simulink model "test"  (R2021a)
settings: Solver=VariableStepAuto  StartTime=0.0  StopTime=60000  RelTol=1e-3
undefined symbols (not defined in the file): Ion, Lithium
libraries: spsSeriesRLCBranchLib x25, spsBatteryLib x20, spsIGBTLib x20, spsIdealSwitchLib x10, spsDCVoltageSourceLib x5, spspowerguiLib x1
settings Model: SimulationMode=rapid-accelerator  Creator=jafar  LastModifiedBy=jafar

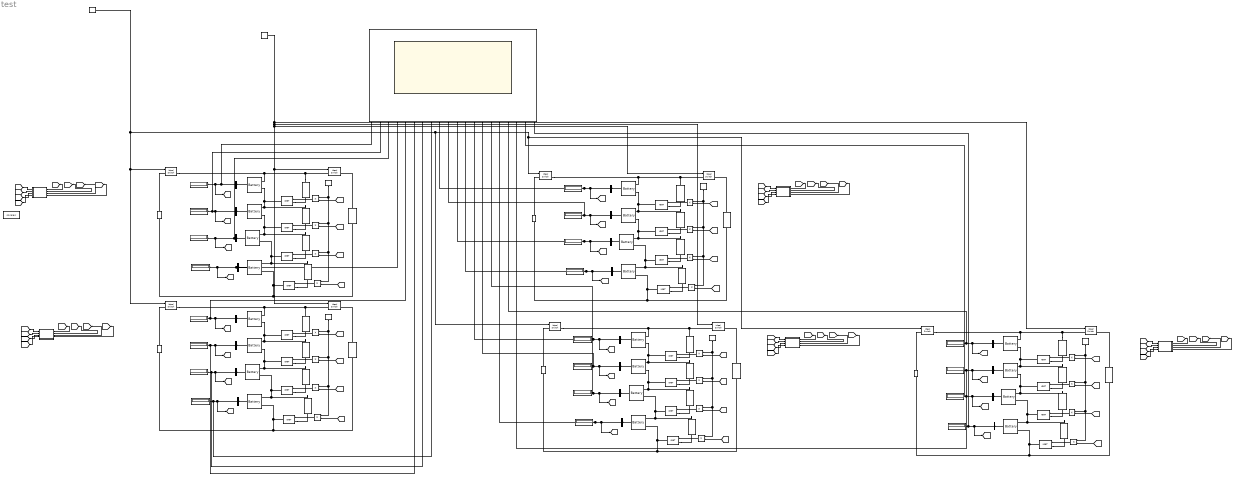
== system test ==
  Battery : spsBatteryLib/Battery  BatType=Lithium-Ion  ShowTempParam=off  ThermalPreset=no  ShowAgeParam=off  NomV=3.7  NomQ=30  SOC=20  Batt_Tr=30  PresetModel=on  MaxQ=30  MinV=2.775  FullV=4.3068  Dis_rate=13.0435  R=0.0012333  Normal_OP=27.1304  expZone="[3.9974      1.4739]"  current=[6.5 13 32.5]  Units=Time  Tci=20  NomT=20  T2=-30  MaxQ2=4.8  FullV2=7.1  Normal_OP2=5.655  expZone2="[6.58           1]"  Rca=0.6  ti=2000  Dp=0  Neq0=0  Tsim=1e6  Ta1=25  Qeol=5.4*0.9  Reol=0.013333*1.2  Char_age=[2.3478, 3]  Dis_age=[2.3478, 10]  N1=1500  N2=10500  N3=1000  N4=1400  Ta2=45  N5=950
  Battery1 : spsBatteryLib/Battery  BatType=Lithium-Ion  ShowTempParam=off  ThermalPreset=no  ShowAgeParam=off  NomV=3.7  NomQ=30  SOC=23  Batt_Tr=30  PresetModel=on  MaxQ=30  MinV=2.775  FullV=4.3068  Dis_rate=13.0435  R=0.0012333  Normal_OP=27.1304  expZone="[3.9974      1.4739]"  current=[6.5 13 32.5]  Units=Time  Tci=20  NomT=20  T2=-30  MaxQ2=4.8  FullV2=7.1  Normal_OP2=5.655  expZone2="[6.58           1]"  Rca=0.6  ti=2000  Dp=0  Neq0=0  Tsim=1e6  Ta1=25  Qeol=5.4*0.9  Reol=0.013333*1.2  Char_age=[2.3478, 3]  Dis_age=[2.3478, 10]  N1=1500  N2=10500  N3=1000  N4=1400  Ta2=45  N5=950
  Battery10 : spsBatteryLib/Battery  BatType=Lithium-Ion  ShowTempParam=off  ThermalPreset=no  ShowAgeParam=off  NomV=3.7  NomQ=30  SOC=60  Batt_Tr=30  PresetModel=on  MaxQ=30  MinV=2.775  FullV=4.3068  Dis_rate=13.0435  R=0.0012333  Normal_OP=27.1304  expZone="[3.9974      1.4739]"  current=[6.5 13 32.5]  Units=Time  Tci=20  NomT=20  T2=-30  MaxQ2=4.8  FullV2=7.1  Normal_OP2=5.655  expZone2="[6.58           1]"  Rca=0.6  ti=2000  Dp=0  Neq0=0  Tsim=1e6  Ta1=25  Qeol=5.4*0.9  Reol=0.013333*1.2  Char_age=[2.3478, 3]  Dis_age=[2.3478, 10]  N1=1500  N2=10500  N3=1000  N4=1400  Ta2=45  N5=950
  Battery11 : spsBatteryLib/Battery  BatType=Lithium-Ion  ShowTempParam=off  ThermalPreset=no  ShowAgeParam=off  NomV=3.7  NomQ=30  SOC=63  Batt_Tr=30  PresetModel=on  MaxQ=30  MinV=2.775  FullV=4.3068  Dis_rate=13.0435  R=0.0012333  Normal_OP=27.1304  expZone="[3.9974      1.4739]"  current=[6.5 13 32.5]  Units=Time  Tci=20  NomT=20  T2=-30  MaxQ2=4.8  FullV2=7.1  Normal_OP2=5.655  expZone2="[6.58           1]"  Rca=0.6  ti=2000  Dp=0  Neq0=0  Tsim=1e6  Ta1=25  Qeol=5.4*0.9  Reol=0.013333*1.2  Char_age=[2.3478, 3]  Dis_age=[2.3478, 10]  N1=1500  N2=10500  N3=1000  N4=1400  Ta2=45  N5=950
  Battery12 : spsBatteryLib/Battery  BatType=Lithium-Ion  ShowTempParam=off  ThermalPreset=no  ShowAgeParam=off  NomV=3.7  NomQ=30  SOC=66  Batt_Tr=30  PresetModel=on  MaxQ=30  MinV=2.775  FullV=4.3068  Dis_rate=13.0435  R=0.0012333  Normal_OP=27.1304  expZone="[3.9974      1.4739]"  current=[6.5 13 32.5]  Units=Time  Tci=20  NomT=20  T2=-30  MaxQ2=4.8  FullV2=7.1  Normal_OP2=5.655  expZone2="[6.58           1]"  Rca=0.6  ti=2000  Dp=0  Neq0=0  Tsim=1e6  Ta1=25  Qeol=5.4*0.9  Reol=0.013333*1.2  Char_age=[2.3478, 3]  Dis_age=[2.3478, 10]  N1=1500  N2=10500  N3=1000  N4=1400  Ta2=45  N5=950
  Battery13 : spsBatteryLib/Battery  BatType=Lithium-Ion  ShowTempParam=off  ThermalPreset=no  ShowAgeParam=off  NomV=3.7  NomQ=30  SOC=69  Batt_Tr=30  PresetModel=on  MaxQ=30  MinV=2.775  FullV=4.3068  Dis_rate=13.0435  R=0.0012333  Normal_OP=27.1304  expZone="[3.9974      1.4739]"  current=[6.5 13 32.5]  Units=Time  Tci=20  NomT=20  T2=-30  MaxQ2=4.8  FullV2=7.1  Normal_OP2=5.655  expZone2="[6.58           1]"  Rca=0.6  ti=2000  Dp=0  Neq0=0  Tsim=1e6  Ta1=25  Qeol=5.4*0.9  Reol=0.013333*1.2  Char_age=[2.3478, 3]  Dis_age=[2.3478, 10]  N1=1500  N2=10500  N3=1000  N4=1400  Ta2=45  N5=950
  Battery14 : spsBatteryLib/Battery  BatType=Lithium-Ion  ShowTempParam=off  ThermalPreset=no  ShowAgeParam=off  NomV=3.7  NomQ=30  SOC=72  Batt_Tr=30  PresetModel=on  MaxQ=30  MinV=2.775  FullV=4.3068  Dis_rate=13.0435  R=0.0012333  Normal_OP=27.1304  expZone="[3.9974      1.4739]"  current=[6.5 13 32.5]  Units=Time  Tci=20  NomT=20  T2=-30  MaxQ2=4.8  FullV2=7.1  Normal_OP2=5.655  expZone2="[6.58           1]"  Rca=0.6  ti=2000  Dp=0  Neq0=0  Tsim=1e6  Ta1=25  Qeol=5.4*0.9  Reol=0.013333*1.2  Char_age=[2.3478, 3]  Dis_age=[2.3478, 10]  N1=1500  N2=10500  N3=1000  N4=1400  Ta2=45  N5=950
  Battery15 : spsBatteryLib/Battery  BatType=Lithium-Ion  ShowTempParam=off  ThermalPreset=no  ShowAgeParam=off  NomV=3.7  NomQ=30  SOC=75  Batt_Tr=30  PresetModel=on  MaxQ=30  MinV=2.775  FullV=4.3068  Dis_rate=13.0435  R=0.0012333  Normal_OP=27.1304  expZone="[3.9974      1.4739]"  current=[6.5 13 32.5]  Units=Time  Tci=20  NomT=20  T2=-30  MaxQ2=4.8  FullV2=7.1  Normal_OP2=5.655  expZone2="[6.58           1]"  Rca=0.6  ti=2000  Dp=0  Neq0=0  Tsim=1e6  Ta1=25  Qeol=5.4*0.9  Reol=0.013333*1.2  Char_age=[2.3478, 3]  Dis_age=[2.3478, 10]  N1=1500  N2=10500  N3=1000  N4=1400  Ta2=45  N5=950
  Battery16 : spsBatteryLib/Battery  BatType=Lithium-Ion  ShowTempParam=off  ThermalPreset=no  ShowAgeParam=off  NomV=3.7  NomQ=30  SOC=78  Batt_Tr=30  PresetModel=on  MaxQ=30  MinV=2.775  FullV=4.3068  Dis_rate=13.0435  R=0.0012333  Normal_OP=27.1304  expZone="[3.9974      1.4739]"  current=[6.5 13 32.5]  Units=Time  Tci=20  NomT=20  T2=-30  MaxQ2=4.8  FullV2=7.1  Normal_OP2=5.655  expZone2="[6.58           1]"  Rca=0.6  ti=2000  Dp=0  Neq0=0  Tsim=1e6  Ta1=25  Qeol=5.4*0.9  Reol=0.013333*1.2  Char_age=[2.3478, 3]  Dis_age=[2.3478, 10]  N1=1500  N2=10500  N3=1000  N4=1400  Ta2=45  N5=950
  Battery17 : spsBatteryLib/Battery  BatType=Lithium-Ion  ShowTempParam=off  ThermalPreset=no  ShowAgeParam=off  NomV=3.7  NomQ=30  SOC=32  Batt_Tr=30  PresetModel=on  MaxQ=30  MinV=2.775  FullV=4.3068  Dis_rate=13.0435  R=0.0012333  Normal_OP=27.1304  expZone="[3.9974      1.4739]"  current=[6.5 13 32.5]  Units=Time  Tci=20  NomT=20  T2=-30  MaxQ2=4.8  FullV2=7.1  Normal_OP2=5.655  expZone2="[6.58           1]"  Rca=0.6  ti=2000  Dp=0  Neq0=0  Tsim=1e6  Ta1=25  Qeol=5.4*0.9  Reol=0.013333*1.2  Char_age=[2.3478, 3]  Dis_age=[2.3478, 10]  N1=1500  N2=10500  N3=1000  N4=1400  Ta2=45  N5=950
  Battery18 : spsBatteryLib/Battery  BatType=Lithium-Ion  ShowTempParam=off  ThermalPreset=no  ShowAgeParam=off  NomV=3.7  NomQ=30  SOC=35  Batt_Tr=30  PresetModel=on  MaxQ=30  MinV=2.775  FullV=4.3068  Dis_rate=13.0435  R=0.0012333  Normal_OP=27.1304  expZone="[3.9974      1.4739]"  current=[6.5 13 32.5]  Units=Time  Tci=20  NomT=20  T2=-30  MaxQ2=4.8  FullV2=7.1  Normal_OP2=5.655  expZone2="[6.58           1]"  Rca=0.6  ti=2000  Dp=0  Neq0=0  Tsim=1e6  Ta1=25  Qeol=5.4*0.9  Reol=0.013333*1.2  Char_age=[2.3478, 3]  Dis_age=[2.3478, 10]  N1=1500  N2=10500  N3=1000  N4=1400  Ta2=45  N5=950
  Battery19 : spsBatteryLib/Battery  BatType=Lithium-Ion  ShowTempParam=off  ThermalPreset=no  ShowAgeParam=off  NomV=3.7  NomQ=30  SOC=38  Batt_Tr=30  PresetModel=on  MaxQ=30  MinV=2.775  FullV=4.3068  Dis_rate=13.0435  R=0.0012333  Normal_OP=27.1304  expZone="[3.9974      1.4739]"  current=[6.5 13 32.5]  Units=Time  Tci=20  NomT=20  T2=-30  MaxQ2=4.8  FullV2=7.1  Normal_OP2=5.655  expZone2="[6.58           1]"  Rca=0.6  ti=2000  Dp=0  Neq0=0  Tsim=1e6  Ta1=25  Qeol=5.4*0.9  Reol=0.013333*1.2  Char_age=[2.3478, 3]  Dis_age=[2.3478, 10]  N1=1500  N2=10500  N3=1000  N4=1400  Ta2=45  N5=950
  Battery2 : spsBatteryLib/Battery  BatType=Lithium-Ion  ShowTempParam=off  ThermalPreset=no  ShowAgeParam=off  NomV=3.7  NomQ=30  SOC=26  Batt_Tr=30  PresetModel=on  MaxQ=30  MinV=2.775  FullV=4.3068  Dis_rate=13.0435  R=0.0012333  Normal_OP=27.1304  expZone="[3.9974      1.4739]"  current=[6.5 13 32.5]  Units=Time  Tci=20  NomT=20  T2=-30  MaxQ2=4.8  FullV2=7.1  Normal_OP2=5.655  expZone2="[6.58           1]"  Rca=0.6  ti=2000  Dp=0  Neq0=0  Tsim=1e6  Ta1=25  Qeol=5.4*0.9  Reol=0.013333*1.2  Char_age=[2.3478, 3]  Dis_age=[2.3478, 10]  N1=1500  N2=10500  N3=1000  N4=1400  Ta2=45  N5=950
  Battery3 : spsBatteryLib/Battery  BatType=Lithium-Ion  ShowTempParam=off  ThermalPreset=no  ShowAgeParam=off  NomV=3.7  NomQ=30  SOC=29  Batt_Tr=30  PresetModel=on  MaxQ=30  MinV=2.775  FullV=4.3068  Dis_rate=13.0435  R=0.0012333  Normal_OP=27.1304  expZone="[3.9974      1.4739]"  current=[6.5 13 32.5]  Units=Time  Tci=20  NomT=20  T2=-30  MaxQ2=4.8  FullV2=7.1  Normal_OP2=5.655  expZone2="[6.58           1]"  Rca=0.6  ti=2000  Dp=0  Neq0=0  Tsim=1e6  Ta1=25  Qeol=5.4*0.9  Reol=0.013333*1.2  Char_age=[2.3478, 3]  Dis_age=[2.3478, 10]  N1=1500  N2=10500  N3=1000  N4=1400  Ta2=45  N5=950
  Battery4 : spsBatteryLib/Battery  BatType=Lithium-Ion  ShowTempParam=off  ThermalPreset=no  ShowAgeParam=off  NomV=3.7  NomQ=30  SOC=42  Batt_Tr=30  PresetModel=on  MaxQ=30  MinV=2.775  FullV=4.3068  Dis_rate=13.0435  R=0.0012333  Normal_OP=27.1304  expZone="[3.9974      1.4739]"  current=[6.5 13 32.5]  Units=Time  Tci=20  NomT=20  T2=-30  MaxQ2=4.8  FullV2=7.1  Normal_OP2=5.655  expZone2="[6.58           1]"  Rca=0.6  ti=2000  Dp=0  Neq0=0  Tsim=1e6  Ta1=25  Qeol=5.4*0.9  Reol=0.013333*1.2  Char_age=[2.3478, 3]  Dis_age=[2.3478, 10]  N1=1500  N2=10500  N3=1000  N4=1400  Ta2=45  N5=950
  Battery5 : spsBatteryLib/Battery  BatType=Lithium-Ion  ShowTempParam=off  ThermalPreset=no  ShowAgeParam=off  NomV=3.7  NomQ=30  SOC=45  Batt_Tr=30  PresetModel=on  MaxQ=30  MinV=2.775  FullV=4.3068  Dis_rate=13.0435  R=0.0012333  Normal_OP=27.1304  expZone="[3.9974      1.4739]"  current=[6.5 13 32.5]  Units=Time  Tci=20  NomT=20  T2=-30  MaxQ2=4.8  FullV2=7.1  Normal_OP2=5.655  expZone2="[6.58           1]"  Rca=0.6  ti=2000  Dp=0  Neq0=0  Tsim=1e6  Ta1=25  Qeol=5.4*0.9  Reol=0.013333*1.2  Char_age=[2.3478, 3]  Dis_age=[2.3478, 10]  N1=1500  N2=10500  N3=1000  N4=1400  Ta2=45  N5=950
  Battery6 : spsBatteryLib/Battery  BatType=Lithium-Ion  ShowTempParam=off  ThermalPreset=no  ShowAgeParam=off  NomV=3.7  NomQ=30  SOC=48  Batt_Tr=30  PresetModel=on  MaxQ=30  MinV=2.775  FullV=4.3068  Dis_rate=13.0435  R=0.0012333  Normal_OP=27.1304  expZone="[3.9974      1.4739]"  current=[6.5 13 32.5]  Units=Time  Tci=20  NomT=20  T2=-30  MaxQ2=4.8  FullV2=7.1  Normal_OP2=5.655  expZone2="[6.58           1]"  Rca=0.6  ti=2000  Dp=0  Neq0=0  Tsim=1e6  Ta1=25  Qeol=5.4*0.9  Reol=0.013333*1.2  Char_age=[2.3478, 3]  Dis_age=[2.3478, 10]  N1=1500  N2=10500  N3=1000  N4=1400  Ta2=45  N5=950
  Battery7 : spsBatteryLib/Battery  BatType=Lithium-Ion  ShowTempParam=off  ThermalPreset=no  ShowAgeParam=off  NomV=3.7  NomQ=30  SOC=51  Batt_Tr=30  PresetModel=on  MaxQ=30  MinV=2.775  FullV=4.3068  Dis_rate=13.0435  R=0.0012333  Normal_OP=27.1304  expZone="[3.9974      1.4739]"  current=[6.5 13 32.5]  Units=Time  Tci=20  NomT=20  T2=-30  MaxQ2=4.8  FullV2=7.1  Normal_OP2=5.655  expZone2="[6.58           1]"  Rca=0.6  ti=2000  Dp=0  Neq0=0  Tsim=1e6  Ta1=25  Qeol=5.4*0.9  Reol=0.013333*1.2  Char_age=[2.3478, 3]  Dis_age=[2.3478, 10]  N1=1500  N2=10500  N3=1000  N4=1400  Ta2=45  N5=950
  Battery8 : spsBatteryLib/Battery  BatType=Lithium-Ion  ShowTempParam=off  ThermalPreset=no  ShowAgeParam=off  NomV=3.7  NomQ=30  SOC=54  Batt_Tr=30  PresetModel=on  MaxQ=30  MinV=2.775  FullV=4.3068  Dis_rate=13.0435  R=0.0012333  Normal_OP=27.1304  expZone="[3.9974      1.4739]"  current=[6.5 13 32.5]  Units=Time  Tci=20  NomT=20  T2=-30  MaxQ2=4.8  FullV2=7.1  Normal_OP2=5.655  expZone2="[6.58           1]"  Rca=0.6  ti=2000  Dp=0  Neq0=0  Tsim=1e6  Ta1=25  Qeol=5.4*0.9  Reol=0.013333*1.2  Char_age=[2.3478, 3]  Dis_age=[2.3478, 10]  N1=1500  N2=10500  N3=1000  N4=1400  Ta2=45  N5=950
  Battery9 : spsBatteryLib/Battery  BatType=Lithium-Ion  ShowTempParam=off  ThermalPreset=no  ShowAgeParam=off  NomV=3.7  NomQ=30  SOC=57  Batt_Tr=30  PresetModel=on  MaxQ=30  MinV=2.775  FullV=4.3068  Dis_rate=13.0435  R=0.0012333  Normal_OP=27.1304  expZone="[3.9974      1.4739]"  current=[6.5 13 32.5]  Units=Time  Tci=20  NomT=20  T2=-30  MaxQ2=4.8  FullV2=7.1  Normal_OP2=5.655  expZone2="[6.58           1]"  Rca=0.6  ti=2000  Dp=0  Neq0=0  Tsim=1e6  Ta1=25  Qeol=5.4*0.9  Reol=0.013333*1.2  Char_age=[2.3478, 3]  Dis_age=[2.3478, 10]  N1=1500  N2=10500  N3=1000  N4=1400  Ta2=45  N5=950
  Bus Selector{,1..19} (20 alike) : BusSelector  OutputSignals=SOC (%)
  Constant{2..3,5,8,11,14} (6 alike) : Constant
  Constant13 : Constant  Value=0
  DC Voltage Source{,1..4} (5 alike) : spsDCVoltageSourceLib/DC Voltage Source  Amplitude=16.8  Measurements=None
  Display{,1..19} (20 alike) : Display
  IGBT{,1..19} (20 alike) : spsIGBTLib/IGBT  Ron=0.001  Lon=0  Vf=1  Tf=1e-6  Tt=2e-6  IC=0  Rs=1e5  Cs=inf  Measurements=off
  Ideal Switch{,1..9} (10 alike) : spsIdealSwitchLib/Ideal Switch  Ron=0.001  Lon=0  IC=0  Rs=1e5  Cs=inf  Measurements=on
  MATLAB Function : MATLAB Function  TreatAsAtomicUnit=on
  MATLAB Function1 : MATLAB Function  TreatAsAtomicUnit=on
  MATLAB Function2 : MATLAB Function  TreatAsAtomicUnit=on
  MATLAB Function3 : MATLAB Function  TreatAsAtomicUnit=on
  MATLAB Function4 : MATLAB Function  TreatAsAtomicUnit=on
  Product{,1..19} (20 alike) : Product
  Scope : Scope  NumInputPorts=20
  Series RLC Branch{,1..24} (25 alike) : spsSeriesRLCBranchLib/Series RLC Branch  LConnTagsString=__new0  RConnTagsString=__new0  BranchType=R  Resistance=1  Inductance=1e-3  SetiL0=off  InitialCurrent=0  Capacitance=1e-6  Setx0=off  InitialVoltage=0  Measurements=None
  powergui : spspowerguiLib/powergui  Priority=1  SimulationMode=Continuous  SampleTime=50e-6  frequency=60  Iterations=50  frequencyindice=0  Pbase=100e6  ErrMax=1e-4  UnitsV=kV  UnitsW=MW  buscounter=0  FunctionMessages=off  echomessages=off  EnableUseOfTLC=off  CurrentSourceSwitches=off  DisableSnubberDevices=off  DisableRonSwitches=off  DisableVfSwitches=off  DisplayEquations=off  AutomaticDiscreteSolvers=off  SolverType=Tustin/Backward Euler (TBE)  Interpol=off  ExternalGateDelay=off  methode=off  Ts=100  x0status=blocks  SPID=on  SwTol=0  HookPort=off  NonlinearTolerance=1e-4  nMaxIteration=100  ContinueOnMaxIteration=off  RestoreLinks=warning  ResistiveCurrentMeasurement=off  Frange=[0:2:500]  Ylog=off  Xlog=on  ShowGrid=off  save=off  variable=ZData  structure=0  ZoomFFT=off  StartTime=0.0  cycles=1  DisplayStyle=1  fundamental=60  FreqAxis=off  MaxFrequency=1000  frequencyindicesteady=1  RmsSteady=1  display=off
  wires:
  [g3] -> Product2/2
  Battery/1 -> Bus Selector/1
  Product2/1 -> IGBT/1
  [g2] -> Product1/2
  Bus Selector1/1 -> [SoC2], Display1/1, Scope/2  "<SOC (%)>"
  Product1/1 -> IGBT1/1
  [g1] -> Product/2
  Product/1 -> IGBT2/1
  Battery2/1 -> Bus Selector2/1
  Battery1/1 -> Bus Selector1/1
  Bus Selector/1 -> Display/1, [SoC1], Scope/1  "<SOC (%)>"
  Bus Selector2/1 -> Display2/1, [SoC3], Scope/3  "<SOC (%)>"
  Bus Selector3/1 -> Display3/1, [SoC4], Scope/4  "<SOC (%)>"
  Battery3/1 -> Bus Selector3/1
  Product3/1 -> IGBT3/1
  Constant2/1 -> Product/1, Product1/1, Product3/1, Product2/1
  [g4] -> Product3/2
  [SoC3] -> MATLAB Function/3(u3)
  [SoC2] -> MATLAB Function/2(u2)
  [SoC1] -> MATLAB Function/1(u1)
  MATLAB Function/2(g2) -> [g2]
  MATLAB Function/3(g3) -> [g3]
  MATLAB Function/1(g1) -> [g1]
  [SoC4] -> MATLAB Function/4(u4)
  MATLAB Function/4(g4) -> [g4]
  MATLAB Function1/2(g2) -> [g6]
  [SoC5] -> MATLAB Function1/1(u1)
  [SoC6] -> MATLAB Function1/2(u2)
  [SoC7] -> MATLAB Function1/3(u3)
  MATLAB Function1/3(g3) -> [g7]
  Battery7/1 -> Bus Selector7/1
  Product7/1 -> IGBT7/1
  Bus Selector7/1 -> [SoC8], Scope/8, Display7/1  "<SOC (%)>"
  MATLAB Function1/4(g4) -> [g8]
  Bus Selector6/1 -> [SoC7], Scope/7, Display6/1  "<SOC (%)>"
  Bus Selector4/1 -> [SoC5], Scope/5, Display4/1  "<SOC (%)>"
  Battery5/1 -> Bus Selector5/1
  [SoC8] -> MATLAB Function1/4(u4)
  Battery6/1 -> Bus Selector6/1
  [g5] -> Product4/2
  Product5/1 -> IGBT5/1
  MATLAB Function1/1(g1) -> [g5]
  Bus Selector5/1 -> [SoC6], Scope/6, Display5/1  "<SOC (%)>"
  [g6] -> Product5/2
  Battery4/1 -> Bus Selector4/1
  Constant5/1 -> Product4/1, Product5/1, Product7/1, Product6/1
  [g8] -> Product7/2
  Product6/1 -> IGBT4/1
  [g7] -> Product6/2
  Product4/1 -> IGBT6/1
  MATLAB Function2/2(g2) -> [g10]
  [SoC9] -> MATLAB Function2/1(u1)
  [SoC10] -> MATLAB Function2/2(u2)
  [SoC11] -> MATLAB Function2/3(u3)
  MATLAB Function2/3(g3) -> [g11]
  Battery11/1 -> Bus Selector11/1
  Product11/1 -> IGBT11/1
  Bus Selector11/1 -> [SoC12], Scope/12, Display11/1  "<SOC (%)>"
  MATLAB Function2/4(g4) -> [g12]
  Bus Selector10/1 -> [SoC11], Scope/11, Display10/1  "<SOC (%)>"
  Bus Selector8/1 -> [SoC9], Scope/9, Display8/1  "<SOC (%)>"
  Battery9/1 -> Bus Selector9/1
  [SoC12] -> MATLAB Function2/4(u4)
  Battery10/1 -> Bus Selector10/1
  [g9] -> Product8/2
  Product9/1 -> IGBT9/1
  MATLAB Function2/1(g1) -> [g9]
  Bus Selector9/1 -> [SoC10], Scope/10, Display9/1  "<SOC (%)>"
  [g10] -> Product9/2
  Battery8/1 -> Bus Selector8/1
  Constant8/1 -> Product8/1, Product9/1, Product11/1, Product10/1
  [g12] -> Product11/2
  Product10/1 -> IGBT8/1
  [g11] -> Product10/2
  Product8/1 -> IGBT10/1
  MATLAB Function3/2(g2) -> [g14]
  [SoC13] -> MATLAB Function3/1(u1)
  [SoC14] -> MATLAB Function3/2(u2)
  [SoC15] -> MATLAB Function3/3(u3)
  MATLAB Function3/3(g3) -> [g15]
  Battery15/1 -> Bus Selector15/1
  Product15/1 -> IGBT15/1
  Bus Selector15/1 -> [SoC16], Scope/16, Display15/1  "<SOC (%)>"
  MATLAB Function3/4(g4) -> [g16]
  Bus Selector14/1 -> [SoC15], Scope/15, Display14/1  "<SOC (%)>"
  Bus Selector12/1 -> [SoC13], Scope/13, Display12/1  "<SOC (%)>"
  Battery13/1 -> Bus Selector13/1
  [SoC16] -> MATLAB Function3/4(u4)
  Battery14/1 -> Bus Selector14/1
  [g13] -> Product12/2
  Product13/1 -> IGBT13/1
  MATLAB Function3/1(g1) -> [g13]
  Bus Selector13/1 -> [SoC14], Scope/14, Display13/1  "<SOC (%)>"
  [g14] -> Product13/2
  Battery12/1 -> Bus Selector12/1
  Constant11/1 -> Product12/1, Product13/1, Product15/1, Product14/1
  [g16] -> Product15/2
  Product14/1 -> IGBT12/1
  Constant13/1 -> Ideal Switch7/1, Ideal Switch5/1, Ideal Switch3/1, Ideal Switch1/1, Ideal Switch9/1
  [g15] -> Product14/2
  Product12/1 -> IGBT14/1
  MATLAB Function4/2(g2) -> [g18]
  MATLAB Function4/4(g4) -> [g20]
  Product16/1 -> IGBT18/1
  Product19/1 -> IGBT19/1
  Product18/1 -> IGBT16/1
  Constant3/1 -> Ideal Switch6/1, Ideal Switch8/1, Ideal Switch4/1, Ideal Switch2/1, Ideal Switch/1
  [SoC18] -> MATLAB Function4/2(u2)
  Battery19/1 -> Bus Selector19/1
  Battery17/1 -> Bus Selector17/1
  Bus Selector16/1 -> [SoC17], Scope/17, Display16/1  "<SOC (%)>"
  [g20] -> Product19/2
  Bus Selector18/1 -> [SoC19], Scope/19, Display18/1  "<SOC (%)>"
  MATLAB Function4/3(g3) -> [g19]
  Bus Selector17/1 -> [SoC18], Scope/18, Display17/1  "<SOC (%)>"
  [SoC17] -> MATLAB Function4/1(u1)
  MATLAB Function4/1(g1) -> [g17]
  Product17/1 -> IGBT17/1
  Battery18/1 -> Bus Selector18/1
  Constant14/1 -> Product16/1, Product17/1, Product19/1, Product18/1
  Battery16/1 -> Bus Selector16/1
  [SoC19] -> MATLAB Function4/3(u3)
  [g17] -> Product16/2
  Bus Selector19/1 -> [SoC20], Scope/20, Display19/1  "<SOC (%)>"
  [g18] -> Product17/2
  [g19] -> Product18/2
  [SoC20] -> MATLAB Function4/4(u4)
  connections:
  Series RLC Branch4/LConn1 -- Battery3/LConn1 -- Battery2/LConn2 -- IGBT/RConn1
  Battery1/LConn1 -- Battery/LConn2 -- IGBT2/RConn1 -- Series RLC Branch1/LConn1
  Series RLC Branch2/LConn1 -- Ideal Switch1/LConn1 -- Battery/LConn1 -- Ideal Switch/RConn1
  Battery2/LConn1 -- Battery1/LConn2 -- IGBT1/RConn1 -- Series RLC Branch/LConn1
  IGBT1/LConn1 -- Series RLC Branch1/RConn1
  IGBT/LConn1 -- Series RLC Branch/RConn1
  Series RLC Branch3/LConn1 -- Ideal Switch1/RConn1
  Ideal Switch/LConn1 -- DC Voltage Source/RConn1
  IGBT2/LConn1 -- Series RLC Branch2/RConn1
  Series RLC Branch3/RConn1 -- DC Voltage Source/LConn1 -- IGBT3/RConn1 -- Battery3/LConn2
  IGBT3/LConn1 -- Series RLC Branch4/RConn1
  Battery6/LConn1 -- Battery5/LConn2 -- IGBT5/RConn1 -- Series RLC Branch5/LConn1
  DC Voltage Source1/LConn1 -- Series RLC Branch8/RConn1 -- IGBT7/RConn1 -- Battery7/LConn2
  Battery5/LConn1 -- Battery4/LConn2 -- IGBT6/RConn1 -- Series RLC Branch6/LConn1
  Ideal Switch2/RConn1 -- Battery4/LConn1 -- Ideal Switch3/LConn1 -- Series RLC Branch7/LConn1
  IGBT4/RConn1 -- Battery6/LConn2 -- Battery7/LConn1 -- Series RLC Branch9/LConn1
  IGBT7/LConn1 -- Series RLC Branch9/RConn1
  IGBT6/LConn1 -- Series RLC Branch7/RConn1
  IGBT5/LConn1 -- Series RLC Branch6/RConn1
  Ideal Switch2/LConn1 -- DC Voltage Source1/RConn1
  IGBT4/LConn1 -- Series RLC Branch5/RConn1
  Series RLC Branch8/LConn1 -- Ideal Switch3/RConn1
  Battery10/LConn1 -- Battery9/LConn2 -- IGBT9/RConn1 -- Series RLC Branch10/LConn1
  DC Voltage Source2/LConn1 -- Series RLC Branch13/RConn1 -- IGBT11/RConn1 -- Battery11/LConn2
  Battery9/LConn1 -- Battery8/LConn2 -- IGBT10/RConn1 -- Series RLC Branch11/LConn1
  Ideal Switch4/RConn1 -- Battery8/LConn1 -- Ideal Switch5/LConn1 -- Series RLC Branch12/LConn1
  IGBT8/RConn1 -- Battery10/LConn2 -- Battery11/LConn1 -- Series RLC Branch14/LConn1
  IGBT11/LConn1 -- Series RLC Branch14/RConn1
  IGBT10/LConn1 -- Series RLC Branch12/RConn1
  IGBT9/LConn1 -- Series RLC Branch11/RConn1
  Ideal Switch4/LConn1 -- DC Voltage Source2/RConn1
  IGBT8/LConn1 -- Series RLC Branch10/RConn1
  Series RLC Branch13/LConn1 -- Ideal Switch5/RConn1
  Battery14/LConn1 -- Battery13/LConn2 -- IGBT13/RConn1 -- Series RLC Branch15/LConn1
  DC Voltage Source3/LConn1 -- Series RLC Branch18/RConn1 -- IGBT15/RConn1 -- Battery15/LConn2
  Battery13/LConn1 -- Battery12/LConn2 -- IGBT14/RConn1 -- Series RLC Branch16/LConn1
  Ideal Switch6/RConn1 -- Battery12/LConn1 -- Ideal Switch7/LConn1 -- Series RLC Branch17/LConn1
  IGBT12/RConn1 -- Battery14/LConn2 -- Battery15/LConn1 -- Series RLC Branch19/LConn1
  IGBT15/LConn1 -- Series RLC Branch19/RConn1
  IGBT14/LConn1 -- Series RLC Branch17/RConn1
  IGBT13/LConn1 -- Series RLC Branch16/RConn1
  Ideal Switch6/LConn1 -- DC Voltage Source3/RConn1
  IGBT12/LConn1 -- Series RLC Branch15/RConn1
  Series RLC Branch18/LConn1 -- Ideal Switch7/RConn1
  DC Voltage Source4/LConn1 -- Series RLC Branch23/RConn1 -- IGBT19/RConn1 -- Battery19/LConn2
  Battery18/LConn1 -- Battery17/LConn2 -- IGBT17/RConn1 -- Series RLC Branch20/LConn1
  Battery17/LConn1 -- Series RLC Branch21/LConn1 -- Battery16/LConn2 -- IGBT18/RConn1
  Series RLC Branch22/LConn1 -- Ideal Switch9/LConn1 -- Battery16/LConn1 -- Ideal Switch8/RConn1
  Series RLC Branch24/LConn1 -- Battery19/LConn1 -- Battery18/LConn2 -- IGBT16/RConn1
  IGBT17/LConn1 -- Series RLC Branch21/RConn1
  IGBT16/LConn1 -- Series RLC Branch20/RConn1
  Ideal Switch8/LConn1 -- DC Voltage Source4/RConn1
  IGBT18/LConn1 -- Series RLC Branch22/RConn1
  IGBT19/LConn1 -- Series RLC Branch24/RConn1
  Series RLC Branch23/LConn1 -- Ideal Switch9/RConn1

== matlab function test/MATLAB Function1 ==
  data: u1 input; g1 output; u2 input; u3 input; g2 output; g3 output; u4 input; g4 output
function [g1,g2,g3,g4] = fcn(u1,u2,u3,u4)

u1 = u1*1000;
u2 = u2*1000;
u3 = u3*1000;
u4 = u4*1000;

u1 = int32(u1);
u2 = int32(u2);
u3 = int32(u3);
u4 = int32(u4);

if u1>u2||u1>u3||u1>u4
    g1 = 1;
else
    g1 = 0;
end
    
if u2>u1||u2>u3||u2>u4
    g2 = 1;
else
    g2 = 0;
end

if u3>u1||u3>u2||u2>u4
    g3 = 1;
else
    g3 = 0;
end
if u4>u1||u4>u2||u4>u3
    g4 = 1;
else
    g4 = 0;
end

end

== matlab function test/MATLAB Function ==
  data: u1 input; g1 output; u2 input; u3 input; g2 output; g3 output; u4 input; g4 output
function [g1,g2,g3,g4] = fcn(u1,u2,u3,u4)

u1 = u1*1000;
u2 = u2*1000;
u3 = u3*1000;
u4 = u4*1000;

u1 = int32(u1);
u2 = int32(u2);
u3 = int32(u3);
u4 = int32(u4);

if u1>u2||u1>u3||u1>u4
    g1 = 1;
else
    g1 = 0;
end
    
if u2>u1||u2>u3||u2>u4
    g2 = 1;
else
    g2 = 0;
end

if u3>u1||u3>u2||u2>u4
    g3 = 1;
else
    g3 = 0;
end
if u4>u1||u4>u2||u4>u3
    g4 = 1;
else
    g4 = 0;
end

end

== matlab function test/MATLAB Function2 ==
  data: u1 input; g1 output; u2 input; u3 input; g2 output; g3 output; u4 input; g4 output
function [g1,g2,g3,g4] = fcn(u1,u2,u3,u4)

u1 = u1*1000;
u2 = u2*1000;
u3 = u3*1000;
u4 = u4*1000;

u1 = int32(u1);
u2 = int32(u2);
u3 = int32(u3);
u4 = int32(u4);

if u1>u2||u1>u3||u1>u4
    g1 = 1;
else
    g1 = 0;
end
    
if u2>u1||u2>u3||u2>u4
    g2 = 1;
else
    g2 = 0;
end

if u3>u1||u3>u2||u2>u4
    g3 = 1;
else
    g3 = 0;
end
if u4>u1||u4>u2||u4>u3
    g4 = 1;
else
    g4 = 0;
end

end

== matlab function test/MATLAB Function3 ==
  data: u1 input; g1 output; u2 input; u3 input; g2 output; g3 output; u4 input; g4 output
function [g1,g2,g3,g4] = fcn(u1,u2,u3,u4)

u1 = u1*1000;
u2 = u2*1000;
u3 = u3*1000;
u4 = u4*1000;

u1 = int32(u1);
u2 = int32(u2);
u3 = int32(u3);
u4 = int32(u4);

if u1>u2||u1>u3||u1>u4
    g1 = 1;
else
    g1 = 0;
end
    
if u2>u1||u2>u3||u2>u4
    g2 = 1;
else
    g2 = 0;
end

if u3>u1||u3>u2||u2>u4
    g3 = 1;
else
    g3 = 0;
end
if u4>u1||u4>u2||u4>u3
    g4 = 1;
else
    g4 = 0;
end

end

== matlab function test/MATLAB Function4 ==
  data: u1 input; g1 output; u2 input; u3 input; g2 output; g3 output; u4 input; g4 output
function [g1,g2,g3,g4] = fcn(u1,u2,u3,u4)

u1 = u1*1000;
u2 = u2*1000;
u3 = u3*1000;
u4 = u4*1000;

u1 = int32(u1);
u2 = int32(u2);
u3 = int32(u3);
u4 = int32(u4);

if u1>u2||u1>u3||u1>u4
    g1 = 1;
else
    g1 = 0;
end
    
if u2>u1||u2>u3||u2>u4
    g2 = 1;
else
    g2 = 0;
end

if u3>u1||u3>u2||u2>u4
    g3 = 1;
else
    g3 = 0;
end
if u4>u1||u4>u2||u4>u3
    g4 = 1;
else
    g4 = 0;
end

end
